simulink model "state_space_01"  (R2019b)
settings: Solver=VariableStepAuto  StartTime=0.0  StopTime=10.0  RelTol=1e-3
values from neighbouring files (symbols this model uses):
  A = [0 1 0 0; -1 -0.2e1 * (K__e * K__t + b__f * R__m / 0.2e1) * (l__b * (l__b + l__w) * m__b + I__b) / ((I__b * l__w ^ 2 + l__b ^ 2 * (l__w ^ 2 * m__w + I__w)) * m__b + I__b * (l__w ^ 2 * m__w + I__w)) / R__m -m__b ^ 2 * l__b ^ 2 * l__w ^ 2 * g / (((m__w + m__b) * l__w ^ 2 + I__w) * I__b + l__b ^ 2 * m__b * (l__w ^ 2 * m__w + I__w)) 0.2e1 * (K__e * K__t + b__f * R__m / 0.2e1) * (l__b ^ 2 * m__b + m__b ...(+714 chars)    [eom.m]    (also in impl_for_sim.m = [0                  1                0              0; state_space_system.m = [0                  1                0              0)
  B = [0 ; 2 * l__w * K__t * (l__b ^ 2 * m__b + m__b * l__b * l__w + I__b) / (((m__w + m__b) * l__w ^ 2 + I__w) * I__b + l__b ^ 2 * m__b * (l__w ^ 2 * m__w + I__w)) / R__m; 0; -2 * ((m__w + m__b) * l__w ^ 2 + m__b * l__b * l__w + I__w) * K__t / (((l__b ^ 2 * m__w + I__b) * m__b + I__b * m__w) * l__w ^ 2 + I__w * (l__b ^ 2 * m__b + I__b)) / R__m]    [eom.m]    (also in impl_for_sim.m = [0              0; state_space_system.m = [0              0)
  C_sim = eye(4)    [impl_for_sim.m]
  D_sim = zeros(4,2)    [impl_for_sim.m]
  K_d = -0.0868    [impl_for_sim.m]
  K_i = -500    [impl_for_sim.m]
  K_p = -200    [impl_for_sim.m]
undefined symbols (not defined in the file or in its folder): sigbuilder_block
libraries: cstblocks x1, simulink x1
settings Model: Creator=jlosi  LastModifiedBy=jlosi

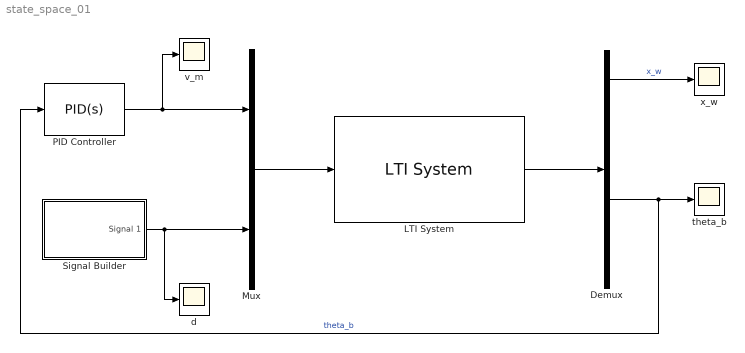
== system state_space_01 ==
  Demux : Demux
  LTI System : cstblocks/LTI System  sys=ss(A,B,C_sim,D_sim)  IC=[]
  Mux : Mux  Inputs=2
  PID Controller : simulink/Continuous/PID Controller  Controller=PID  Form=Parallel  TimeDomain=Continuous-time  SampleTime=-1  IntegratorMethod=Forward Euler  FilterMethod=Forward Euler  ControllerParametersSource=internal  P=-K_p  I=-K_i  D=-K_d  UseFilter=on  N=100  TunerSelectOption=Transfer Function Based (PID Tuner App)  InitialConditionSource=internal  InitialConditionForIntegrator=0  InitialConditionForFilter=0  DifferentiatorICPrevScaledInput=0  ExternalReset=none  TrackingMode=off  Kt=1  LimitOutput=off  UpperSaturationLimit=inf  LowerSaturationLimit=-inf  LinearizeAsGain=on  AntiWindupMode=none  Kb=1  POutMin=[]  POutMax=[]  IOutMin=[]  IOutMax=[]  DOutMin=[]  DOutMax=[]  NOutMin=[]  NOutMax=[]  SumOutMin=[]  SumOutMax=[]  SaturationOutMin=[]  SaturationOutMax=[]  PParamMin=[]  PParamMax=[]  IParamMin=[]  IParamMax=[]  DParamMin=[]  DParamMax=[]  NParamMin=[]  NParamMax=[]  KbParamMin=[]  KbParamMax=[]  KtParamMin=[]  KtParamMax=[]  KbOutMin=[]  KbOutMax=[]  KtOutMin=[]  KtOutMax=[]  IntegratorOutMin=[]  IntegratorOutMax=[]  FilterOutMin=[]  FilterOutMax=[]  SumI1OutMin=[]  SumI1OutMax=[]  SumI2OutMin=[]  SumI2OutMax=[]  SumI3OutMin=[]  SumI3OutMax=[]  SumI4OutMin=[]  SumI4OutMax=[]  SumDOutMin=[]  SumDOutMax=[]  DifferentiatorOutMin=[]  DifferentiatorOutMax=[]  FilterDiffOutCoefMin=[]  FilterDiffOutCoefMax=[]  ReciprocalOutMin=[]  ReciprocalOutMax=[]  SumDenOutMin=[]  SumDenOutMax=[]  SumNumOutMin=[]  SumNumOutMax=[]  DivideOutMin=[]  DivideOutMax=[]  IntegratorContinuousStateAttributes=''  IntegratorStateMustResolveToSignalObject=off  IntegratorRTWStateStorageClass=Auto  FilterContinuousStateAttributes=''  FilterStateMustResolveToSignalObject=off  FilterRTWStateStorageClass=Auto  ParallelPVariant=InternalParameters  IdealPVariant=Disabled  IVariant=InternalParameters  DVariant=InternalParameters  IntegratorVariant=Continuous  SatVariant=Disabled  AWVariant=Passthrough  PCopyVariant=Disabled  TRVariant=Disabled  FdbkBlocksVariant=Forward  IdealPFdbkVariant=Disabled  SatFdbkVariant=Disabled  DerivativeFilterVariant=ContFilter  NVariant=InternalParameters  NCopyVariant=Disabled  FilterICVariant=InternalICsFilter  IntegratorICVariant=InternalICs  ExternalResetVariant=Disabled  TRSumVariant=Passthrough  SumFdbkVariant=Disabled  SumVariant=Sum_PID
  Signal Builder : Subsystem  Tag=STV Subsys  LoadFcn=sigbuilder_block('load',[378.6 18.6 768 458.4 ]);  StartFcn=sigbuilder_block('start');  StopFcn=sigbuilder_block('stop');  ClipboardFcn=sigbuilder_block('clipboard');  mask(Sigbuilder block){tuvar=[0:10]}
      mask help: Simulink:masks:SigbuilderBlock_MD
      mask init:
      | if ~strcmp(get_param(bdroot(gcbh),'SimulationStatus'),'stopped') tuvar = sigbuilder_block('maskInit'); end
      settings: CopyFcn=sigbuilder_block('copy');  DeleteFcn=sigbuilder_block('delete');  ModelCloseFcn=sigbuilder_block('modelClose');  PreSaveFcn=sigbuilder_block('preSave');  PauseFcn=sigbuilder_block('pause');  ContinueFcn=sigbuilder_block('continue');  NameChangeFcn=sigbuilder_block('namechange');  OpenFcn=sigbuilder_block('open',[1582.2 18.6 768 497.4 ]);  CloseFcn=sigbuilder_block('close');
      mask Display: plot(0, 0, 100, 100,[2, 2, 32, 32, 2], [68, 8, 8, 68, 68],[32, 2], [38, 38], [32, 19, 2],[53, 60, 44], [32, 17, 17, 2],[16, 16, 31, 31]);txt = getActiveGroup(gcbh);text(2, 100, txt,'verticalAlignment', 'top');
  d : Scope
  theta_b : Scope
  v_m : Scope
  "x_w " : Scope
  wires:
  Signal Builder/1(Signal 1) -> d/1, Mux/2
  PID Controller/1 -> v_m/1, Mux/1
  Mux/1 -> LTI System/1
  LTI System/1 -> Demux/1
  Demux/1 -> "x_w "/1  "x_w"
  Demux/3 -> PID Controller/1, theta_b/1  "theta_b"

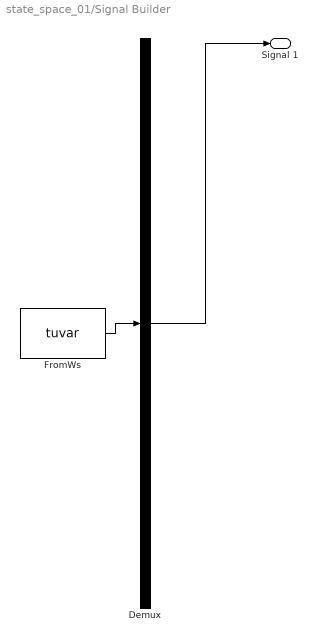
== system state_space_01/Signal Builder ==
  Demux : Demux  Tag=STV Demux  Outputs=1
  FromWs : FromWorkspace  Tag=STV FromWs  VariableName=tuvar  SampleTime=0
      SigBuilderData=|
      | common.afterFinalStr = 'Extrapolate'
      | common.sampleTime = 0
      | dataSet.timeRange = [0 10]
      | dataSet.name = 'Group 1'
      | sbobj.Groups.Name = 'Group 1'
      | sbobj.Groups.Signals.Name = 'Signal 1'
      | sbobj.Groups.Signals.XData = [0 0.1 0.1 6 10]
      | sbobj.Groups.Signals.YData = [0.1 0.1 0 0 0]
  Signal 1 : Outport  Tag=STV Outport
  wires:
  Demux/1 -> Signal 1/1
  FromWs/1 -> Demux/1
